simulink model "simulink_ROS_interface_blocks"  (R2019b)
settings: Solver=FixedStepAuto  StartTime=0.0  StopTime=Inf  FixedStep=FIXED_STEP_SIZE  RelTol=1e-3
undefined symbols (not defined in the file or in its folder): Angular, AngularVelocities, AngularVelocities_SL_Info, FIXED_STEP_SIZE, Header, Linear, Pitch, RAD2DEG, Roll, Thrust, THRUST_OFFSET, YawRate
libraries: robotlib x12, robotgazebolib x1
settings Model: Creator=ananda  LastModifiedBy=ananda

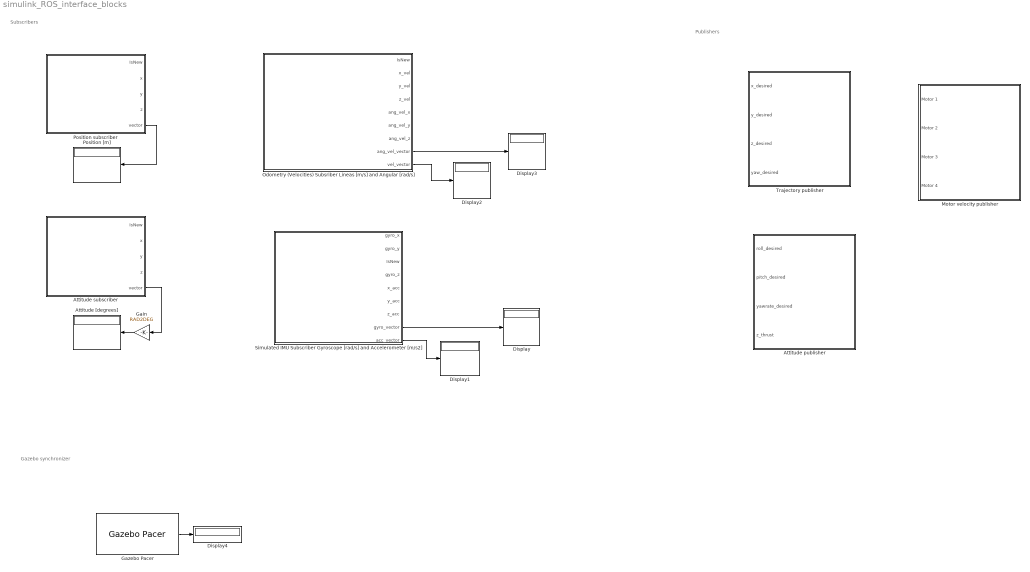
== system simulink_ROS_interface_blocks ==
  note: Gazebo synchronizer
  note: Publishers
  note: Subscribers
  Attitude [degrees] : Display
  Attitude publisher : Subsystem
  Attitude subscriber : Subsystem
  Display{,1..4} (5 alike) : Display
  Gain : Gain  Gain=RAD2DEG
  Gazebo Pacer : robotgazebolib/Gazebo Pacer  ResetBehavior=Reset Gazebo simulation time  SampleTime=FIXED_STEP_SIZE
      settings: SourceProductName=Robotics System Toolbox  SourceProductBaseCode=RO
  Motor velocity publisher : Subsystem
  Odometry (Velocities) Subsriber Lineas [m/s] and Angular [rad/s] : Subsystem
  Position [m] : Display
  Position subscriber : Subsystem
  Simulated IMU Subscriber Gyroscope [rad/s] and Accelerometer [m/s2] : Subsystem
  Trajectory publisher : Subsystem
  wires:
  Position subscriber/5(vector) -> Position [m]/1
  Gain/1 -> Attitude [degrees]/1
  Attitude subscriber/5(vector) -> Gain/1
  Simulated IMU Subscriber Gyroscope [rad/s] and Accelerometer [m/s2]/8(gyro_vector) -> Display/1
  Simulated IMU Subscriber Gyroscope [rad/s] and Accelerometer [m/s2]/9(acc_vector) -> Display1/1
  Odometry (Velocities) Subsriber Lineas [m/s] and Angular [rad/s]/9(vel_vector) -> Display2/1
  Odometry (Velocities) Subsriber Lineas [m/s] and Angular [rad/s]/8(ang_vel_vector) -> Display3/1
  Gazebo Pacer/1 -> Display4/1

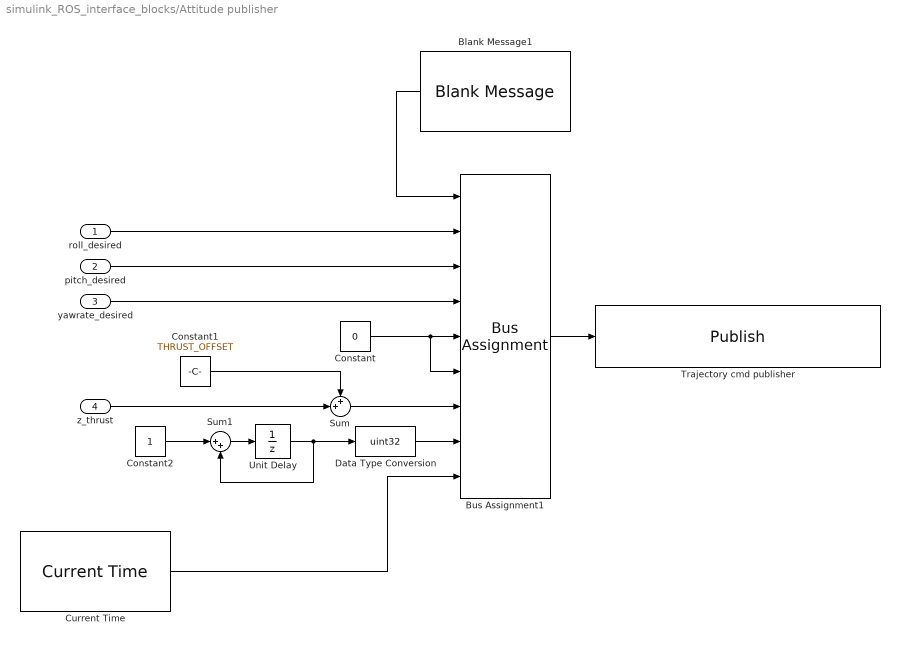
== system simulink_ROS_interface_blocks/Attitude publisher ==
  roll_desired : Inport
  pitch_desired : Inport  Port=2
  yawrate_desired : Inport  Port=3
  z_thrust : Inport  Port=4
  Blank Message1 : robotlib/Blank Message  messageClass=Message  entityType=mav_msgs/RollPitchYawrateThrust  messageType=mav_msgs/RollPitchYawrateThrust  SampleTime=FIXED_STEP_SIZE
      settings: SourceProductName=ROS Toolbox
  Bus Assignment1 : BusAssignment  AssignedSignals=Roll,Pitch,YawRate,Thrust.X,Thrust.Y,Thrust.Z,Header.Seq,Header.Stamp
  Constant : Constant  Value=0
  Constant1 : Constant  Value=THRUST_OFFSET
  Constant2 : Constant
  Current Time : robotlib/Current Time  OutputFormat=bus  SampleTime=FIXED_STEP_SIZE  ModelName=attitude_interface
      settings: SourceProductName=ROS Toolbox  SourceProductBaseCode=RR
  Data Type Conversion : DataTypeConversion  OutDataTypeStr=uint32
  Sum : Sum  Inputs=++|
  Sum1 : Sum  Inputs=|++
  Trajectory cmd publisher : robotlib/Publish  topicSource=Specify your own  topic=/hummingbird/command/roll_pitch_yawrate_thrust  messageType=mav_msgs/RollPitchYawrateThrust  messageQueueLength=1
      settings: SourceProductName=ROS Toolbox
  Unit Delay : UnitDelay  SampleTime=FIXED_STEP_SIZE  HasFrameUpgradeWarning=on
  wires:
  Bus Assignment1/1 -> Trajectory cmd publisher/1
  Blank Message1/1 -> Bus Assignment1/1
  Constant/1 -> Bus Assignment1/6, Bus Assignment1/5
  yawrate_desired/1 -> Bus Assignment1/4
  pitch_desired/1 -> Bus Assignment1/3
  roll_desired/1 -> Bus Assignment1/2
  Sum/1 -> Bus Assignment1/7
  z_thrust/1 -> Sum/2
  Constant1/1 -> Sum/1
  Sum1/1 -> Unit Delay/1
  Unit Delay/1 -> Sum1/2, Data Type Conversion/1
  Constant2/1 -> Sum1/1
  Current Time/1 -> Bus Assignment1/9
  Data Type Conversion/1 -> Bus Assignment1/8

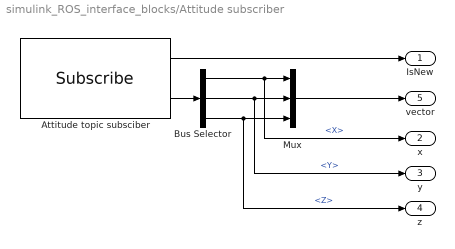
== system simulink_ROS_interface_blocks/Attitude subscriber ==
  Attitude topic subsciber : robotlib/Subscribe  topicSource=Specify your own  topic=/hummingbird/orientation_rpy  messageType=geometry_msgs/Vector3  sampleTime=ATTI_SUB_DT  messageQueueLength=1
      settings: SourceProductName=ROS Toolbox
  Bus Selector : BusSelector  OutputSignals=X,Y,Z
  Mux : Mux  Inputs=3
  IsNew : Outport
  x : Outport  Port=2
  y : Outport  Port=3
  z : Outport  Port=4
  vector : Outport  Port=5
  wires:
  Bus Selector/3 -> z/1, Mux/3  "<Z>"
  Bus Selector/2 -> y/1, Mux/2  "<Y>"
  Bus Selector/1 -> x/1, Mux/1  "<X>"
  Attitude topic subsciber/2 -> Bus Selector/1
  Attitude topic subsciber/1 -> IsNew/1
  Mux/1 -> vector/1

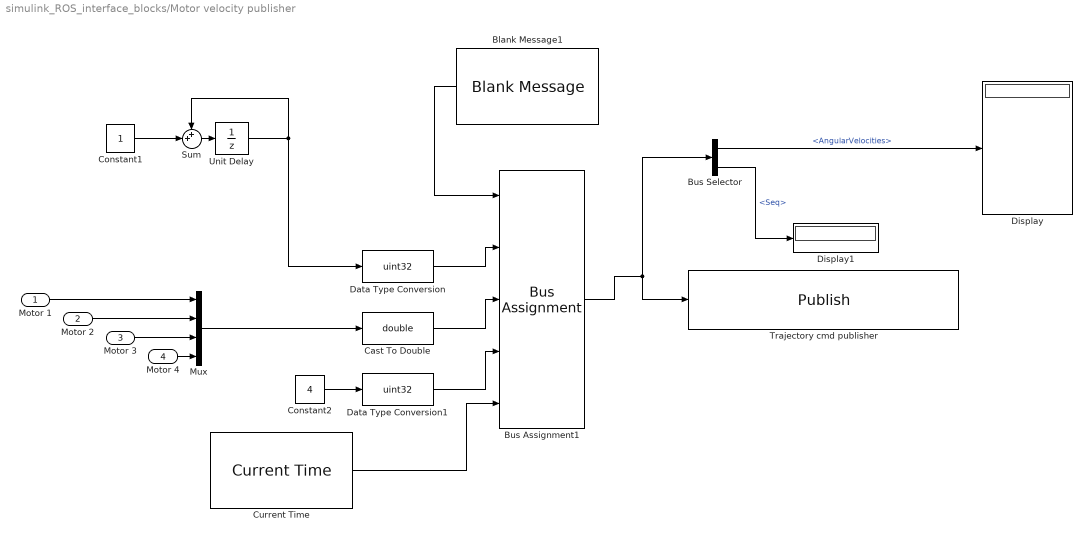
== system simulink_ROS_interface_blocks/Motor velocity publisher ==
  Motor 1 : Inport
  Motor 2 : Inport  Port=2
  Motor 3 : Inport  Port=3
  Motor 4 : Inport  Port=4
  Blank Message1 : robotlib/Blank Message  messageClass=Message  entityType=mav_msgs/Actuators  messageType=mav_msgs/Actuators  SampleTime=inf
      settings: SourceProductName=ROS Toolbox
  Bus Assignment1 : BusAssignment  AssignedSignals=Header.Seq,AngularVelocities,AngularVelocities_SL_Info.CurrentLength,Header.Stamp
  Bus Selector : BusSelector  OutputSignals=AngularVelocities,Header.Seq
  Cast To Double : DataTypeConversion  OutDataTypeStr=double
  Constant1 : Constant
  Constant2 : Constant  Value=4
  Current Time : robotlib/Current Time  OutputFormat=bus  SampleTime=FIXED_STEP_SIZE  ModelName=motor_velocity_interface
      settings: SourceProductName=ROS Toolbox  SourceProductBaseCode=RR
  Data Type Conversion : DataTypeConversion  OutDataTypeStr=uint32
  Data Type Conversion1 : DataTypeConversion  OutDataTypeStr=uint32
  Display : Display
  Display1 : Display
  Mux : Mux
  Sum : Sum  Inputs=++|
  Trajectory cmd publisher : robotlib/Publish  topicSource=Specify your own  topic=/hummingbird/command/motor_speed  messageType=mav_msgs/Actuators  messageQueueLength=1
      settings: SourceProductName=ROS Toolbox
  Unit Delay : UnitDelay  SampleTime=FIXED_STEP_SIZE  HasFrameUpgradeWarning=on
  wires:
  Bus Assignment1/1 -> Trajectory cmd publisher/1, Bus Selector/1
  Blank Message1/1 -> Bus Assignment1/1
  Data Type Conversion/1 -> Bus Assignment1/2
  Mux/1 -> Cast To Double/1
  Cast To Double/1 -> Bus Assignment1/3
  Bus Selector/1 -> Display/1  "<AngularVelocities>"
  Bus Selector/2 -> Display1/1  "<Seq>"
  Constant2/1 -> Data Type Conversion1/1
  Data Type Conversion1/1 -> Bus Assignment1/4
  Motor 1/1 -> Mux/1
  Motor 2/1 -> Mux/2
  Motor 3/1 -> Mux/3
  Motor 4/1 -> Mux/4
  Current Time/1 -> Bus Assignment1/5
  Sum/1 -> Unit Delay/1
  Unit Delay/1 -> Data Type Conversion/1, Sum/1
  Constant1/1 -> Sum/2

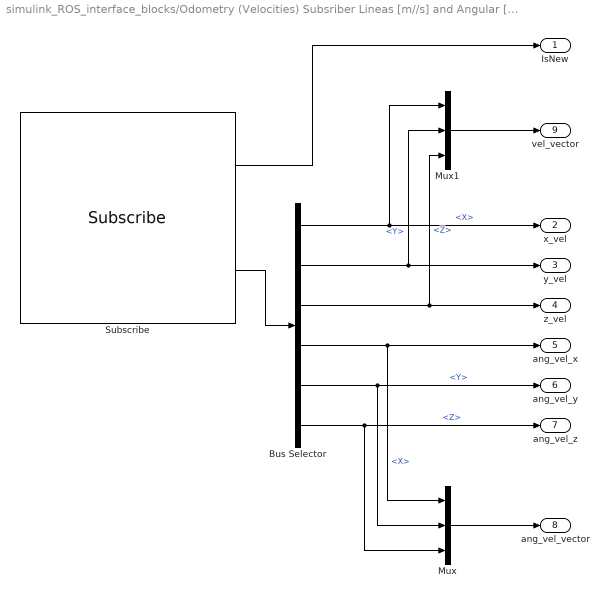
== system simulink_ROS_interface_blocks/Odometry (Velocities) Subsriber Lineas [m//s] and Angular [rad//s] ==
  Bus Selector : BusSelector  OutputSignals=Twist.Twist.Linear.X,Twist.Twist.Linear.Y,Twist.Twist.Linear.Z,Twist.Twist.Angular.X,Twist.Twist.Angular.Y,Twist.Twist.Angular.Z
  Mux : Mux  Inputs=3
  Mux1 : Mux  Inputs=3
  Subscribe : robotlib/Subscribe  topicSource=Specify your own  topic=/hummingbird/odometry_sensor1/odometry  messageType=nav_msgs/Odometry  sampleTime=ODOMETRY_SUB_DT  messageQueueLength=1
      settings: SourceProductName=ROS Toolbox
  IsNew : Outport
  x_vel : Outport  Port=2
  y_vel : Outport  Port=3
  z_vel : Outport  Port=4
  ang_vel_x : Outport  Port=5
  ang_vel_y : Outport  Port=6
  ang_vel_z : Outport  Port=7
  ang_vel_vector : Outport  Port=8
  vel_vector : Outport  Port=9
  wires:
  Bus Selector/4 -> Mux/1, ang_vel_x/1  "<X>"
  Bus Selector/6 -> Mux/3, ang_vel_z/1  "<Z>"
  Bus Selector/2 -> Mux1/2, y_vel/1  "<Y>"
  Subscribe/1 -> IsNew/1
  Bus Selector/5 -> Mux/2, ang_vel_y/1  "<Y>"
  Bus Selector/1 -> Mux1/1, x_vel/1  "<X>"
  Subscribe/2 -> Bus Selector/1
  Bus Selector/3 -> Mux1/3, z_vel/1  "<Z>"
  Mux/1 -> ang_vel_vector/1
  Mux1/1 -> vel_vector/1

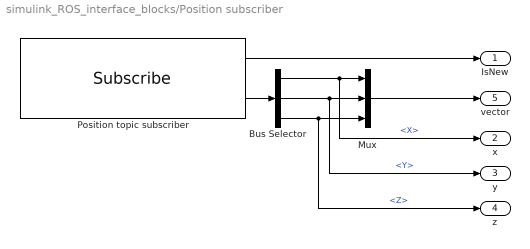
== system simulink_ROS_interface_blocks/Position subscriber ==
  Bus Selector : BusSelector  OutputSignals=Point.X,Point.Y,Point.Z
  Mux : Mux  Inputs=3
  Position topic subscriber : robotlib/Subscribe  topicSource=Specify your own  topic=/hummingbird/odometry_sensor1/position  messageType=geometry_msgs/PointStamped  sampleTime=POS_SUB_DT  messageQueueLength=1
      settings: SourceProductName=ROS Toolbox
  IsNew : Outport
  x : Outport  Port=2
  y : Outport  Port=3
  z : Outport  Port=4
  vector : Outport  Port=5
  wires:
  Bus Selector/3 -> z/1, Mux/3  "<Z>"
  Bus Selector/2 -> y/1, Mux/2  "<Y>"
  Mux/1 -> vector/1
  Bus Selector/1 -> x/1, Mux/1  "<X>"
  Position topic subscriber/2 -> Bus Selector/1
  Position topic subscriber/1 -> IsNew/1

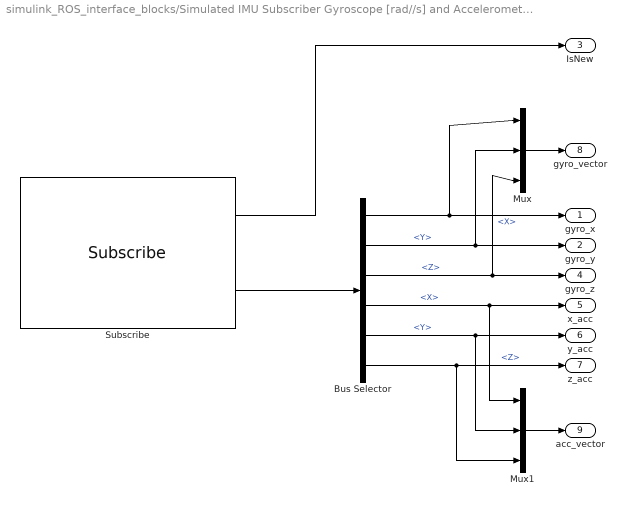
== system simulink_ROS_interface_blocks/Simulated IMU Subscriber Gyroscope [rad//s] and Accelerometer [m//s2] ==
  Bus Selector : BusSelector  OutputSignals=AngularVelocity.X,AngularVelocity.Y,AngularVelocity.Z,LinearAcceleration.X,LinearAcceleration.Y,LinearAcceleration.Z
  Mux : Mux  Inputs=3
  Mux1 : Mux  Inputs=3
  Subscribe : robotlib/Subscribe  topicSource=Specify your own  topic=/hummingbird/imu  messageType=sensor_msgs/Imu  sampleTime=IMU_SUB_DT  messageQueueLength=1
      settings: SourceProductName=ROS Toolbox
  gyro_x : Outport
  gyro_y : Outport  Port=2
  IsNew : Outport  Port=3
  gyro_z : Outport  Port=4
  x_acc : Outport  Port=5
  y_acc : Outport  Port=6
  z_acc : Outport  Port=7
  gyro_vector : Outport  Port=8
  acc_vector : Outport  Port=9
  wires:
  Bus Selector/6 -> Mux1/3, z_acc/1  "<Z>"
  Bus Selector/2 -> Mux/2, gyro_y/1  "<Y>"
  Bus Selector/5 -> Mux1/2, y_acc/1  "<Y>"
  Subscribe/2 -> Bus Selector/1
  Subscribe/1 -> IsNew/1
  Bus Selector/4 -> Mux1/1, x_acc/1  "<X>"
  Bus Selector/3 -> Mux/3, gyro_z/1  "<Z>"
  Bus Selector/1 -> Mux/1, gyro_x/1  "<X>"
  Mux/1 -> gyro_vector/1
  Mux1/1 -> acc_vector/1

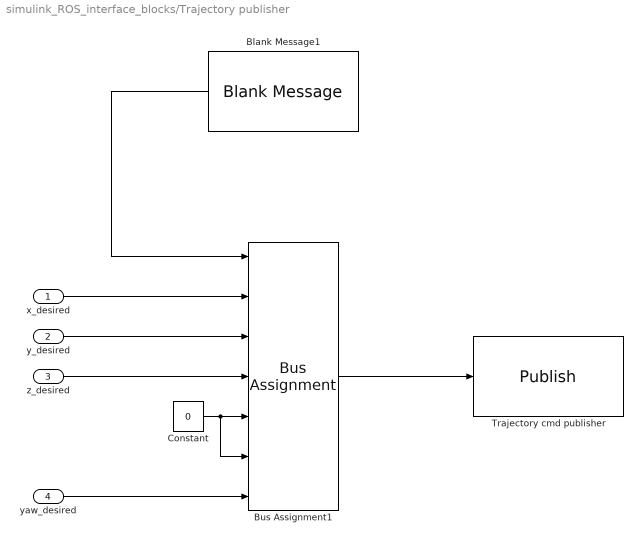
== system simulink_ROS_interface_blocks/Trajectory publisher ==
  x_desired : Inport
  y_desired : Inport  Port=2
  z_desired : Inport  Port=3
  yaw_desired : Inport  Port=4
  Blank Message1 : robotlib/Blank Message  messageClass=Message  entityType=geometry_msgs/Twist  messageType=geometry_msgs/Twist  SampleTime=inf
      settings: SourceProductName=ROS Toolbox
  Bus Assignment1 : BusAssignment  AssignedSignals=Linear.X,Linear.Y,Linear.Z,Angular.X,Angular.Y,Angular.Z
  Constant : Constant  Value=0
  Trajectory cmd publisher : robotlib/Publish  topicSource=Specify your own  topic=/matlab/tracejtoryTwist  messageType=geometry_msgs/Twist  messageQueueLength=1
      settings: SourceProductName=ROS Toolbox
  wires:
  Blank Message1/1 -> Bus Assignment1/1
  Constant/1 -> Bus Assignment1/6, Bus Assignment1/5
  Bus Assignment1/1 -> Trajectory cmd publisher/1
  x_desired/1 -> Bus Assignment1/2
  y_desired/1 -> Bus Assignment1/3
  z_desired/1 -> Bus Assignment1/4
  yaw_desired/1 -> Bus Assignment1/7
